simulink model "Task2"  (R2022a)
settings: Solver=FixedStepAuto  StartTime=0.0  StopTime=2  FixedStep=0.01  RelTol=1e-3
values from neighbouring files (symbols this model uses):
  A = [-3 0 0 ... (first row only)    [Matlabfileassign2.m]
  B = [1 0 0 ... (first row only)    [Matlabfileassign2.m]
  C = [1 0 0 ... (first row only)    [Matlabfileassign2.m]
  F = lqr(A,B,Q,R)    [Matlabfileassign2.m]
  WW = -inv(C*inv(A-B*F)*B)    [Matlabfileassign2.m]
settings Model: Creator=Abdur Rafay  LastModifiedBy=Abdur Rafay

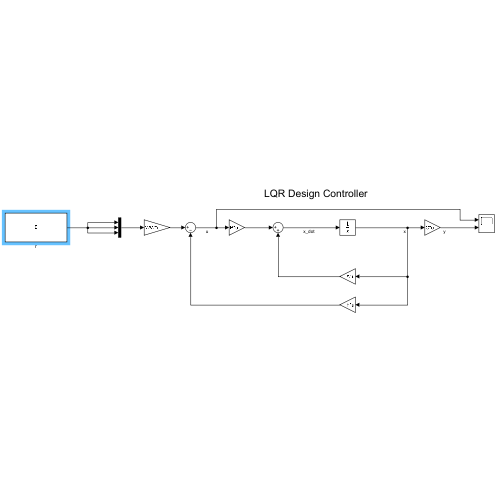
[thumbnail: Simulink's stored preview of the top-level diagram]
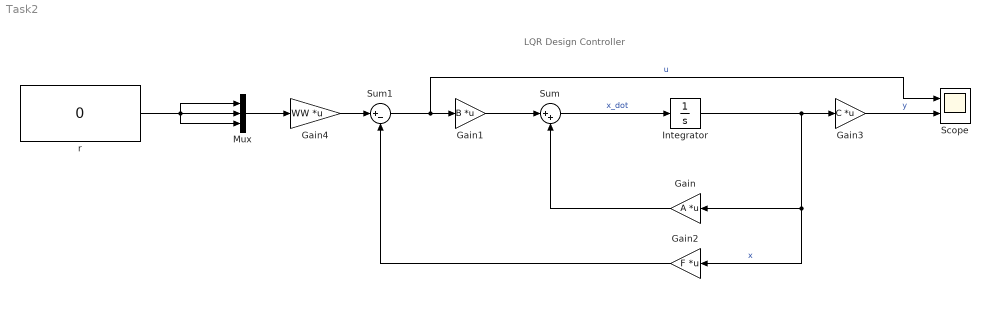
== system Task2 ==
  note: LQR Design Controller
  Gain : Gain  Gain=A  Multiplication=Matrix(K*u)
  Gain1 : Gain  Gain=B  Multiplication=Matrix(K*u)
  Gain2 : Gain  Gain=F  Multiplication=Matrix(K*u)
  Gain3 : Gain  Gain=C  Multiplication=Matrix(K*u)
  Gain4 : Gain  Gain=WW  Multiplication=Matrix(K*u)
  Integrator : Integrator  InitialCondition=[1 1 1]
  Mux : Mux  Inputs=3
  Scope : Scope  NumInputPorts=2
  Sum : Sum  Inputs=|++
  Sum1 : Sum  Inputs=|+-
  r : Constant  Value=0
  wires:
  Sum/1 -> Integrator/1  "x_dot"
  Gain1/1 -> Sum/1
  Gain/1 -> Sum/2
  Integrator/1 -> Gain2/1, Gain/1, Gain3/1  "x"
  Sum1/1 -> Scope/1, Gain1/1  "u"
  Gain2/1 -> Sum1/2
  r/1 -> Mux/1, Mux/3, Mux/2
  Gain4/1 -> Sum1/1
  Mux/1 -> Gain4/1
  Gain3/1 -> Scope/2  "y"
